simulink model "Mahendra_ev"  (R2024a)
settings: Solver=VariableStepAuto  StartTime=0.0  StopTime=100  RelTol=1e-3
undefined symbols (not defined in the file): magnitude
libraries: simulink_extras x1
settings Model: Creator=appu  LastModifiedBy=appu

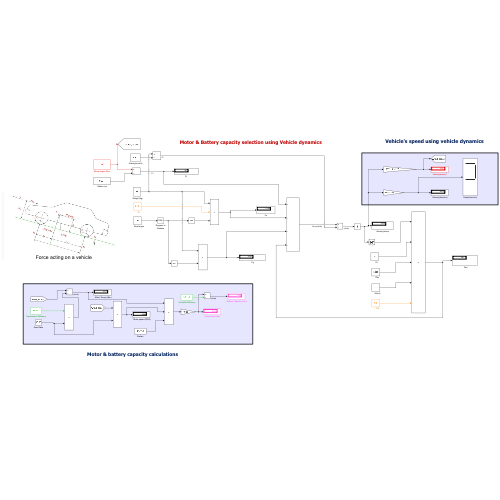
[thumbnail: Simulink's stored preview of the top-level diagram]
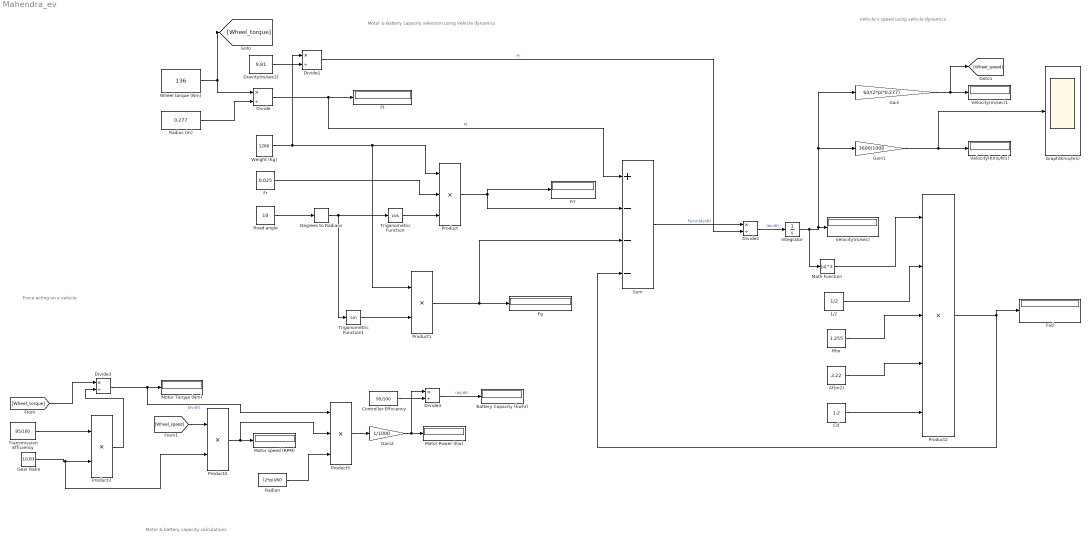
== system Mahendra_ev ==
  note: Force acting on a vehicle
  note: Vehicle's speed using vehicle dynamics
  note: Motor & battery capacity calculations
  note: Motor & Battery capacity selection using Vehicle dynamics
  "       Af(m2)" : Constant  Value=2.22
  "       Cd" : Constant  Value=1.2
  "      1/2" : Constant  Value=1/2
  "      Rho" : Constant  Value=1.255
  "      Road angle" : Constant  Value=10
  "     Fr" : Constant  Value=0.025
  "   Battery Capacity (kwhr)" : Display
  "   Fad" : Display
  "   Motor Torque (Nm)" : Display
  "   Motor speed (RPM)" : Display
  "   Weight (Kg)" : Constant  Value=1260
  "  Fg" : Display
  "  Motor Power (Kw)" : Display
  " Controller Efficiency" : Constant  Value=95/100
  " Frr" : Display
  " Gravity(m/sec2)" : Constant  Value=9.81
  " Radius (m)" : Constant  Value=0.277
  " Velocity(Kms/hrs)" : Display
  " Velocity(m/sec)" : Display
  " Velocity(m/sec)1" : Display
  Degrees to Radians : simulink_extras/Transformations/Degrees to Radians
  Divide{,1..4} (5 alike) : Product  Inputs=*/
  Ft : Display
  Gain : Gain  Gain=60/(2*pi*0.277)
  Gain1 : Gain  Gain=3600/1000
  Gain2 : Gain  Gain=1/1000
  Gear Ratio : Constant  Value=10.83
  Graph(Kms/hrs) : Scope
  Integrator : Integrator
  Math Function : Math  Operator=magnitude^2
  Product : Product  Inputs=3
  Product1 : Product
  Product2 : Product  Inputs=5
  Product3 : Product
  Product4 : Product
  Product5 : Product  Inputs=3
  Radian : Constant  Value=(2*pi)/60
  Sum : Sum  Inputs=+---
  Transmission Efficiency : Constant  Value=85/100
  Trigonometric Function : Trigonometry  Operator=cos
  Trigonometric Function1 : Trigonometry
  Wheel torque (Nm) : Constant  Value=136
  wires:
  Wheel torque (Nm)/1 -> [Wheel_torque], Divide/1
  " Radius (m)"/1 -> Divide/2
  "      Road angle"/1 -> Degrees to Radians/1
  Degrees to Radians/1 -> Trigonometric Function1/1, Trigonometric Function/1
  Trigonometric Function/1 -> Product/3
  "     Fr"/1 -> Product/2
  "   Weight (Kg)"/1 -> Product1/1, Product/1, Divide1/1
  Divide/1 -> Sum/1, Ft/1  "Ft"
  Product/1 -> Sum/2, " Frr"/1
  " Gravity(m/sec2)"/1 -> Divide1/2
  Sum/1 -> Divide2/1  "Fa=m(dv/dt)"
  Divide1/1 -> Divide2/2  "Ft"
  Divide2/1 -> Integrator/1  "(dv/dt)"
  Integrator/1 -> Math Function/1, Gain1/1, Gain/1, " Velocity(m/sec)"/1
  Math Function/1 -> Product2/1
  "      1/2"/1 -> Product2/2
  "      Rho"/1 -> Product2/3
  "       Af(m2)"/1 -> Product2/4
  "       Cd"/1 -> Product2/5
  Gain/1 -> [Wheel_speed], " Velocity(m/sec)1"/1
  Gain1/1 -> Graph(Kms/hrs)/1, " Velocity(Kms/hrs)"/1
  Product2/1 -> Sum/4, "   Fad"/1
  Transmission Efficiency/1 -> Product3/1
  Gear Ratio/1 -> Product4/2, Product3/2
  [Wheel_torque] -> Divide3/1
  Product3/1 -> Divide3/2
  [Wheel_speed] -> Product4/1
  Divide3/1 -> Product5/1, "   Motor Torque (Nm)"/1  "(dv/dt)"
  Product4/1 -> Product5/2, "   Motor speed (RPM)"/1
  Radian/1 -> Product5/3
  Product5/1 -> Gain2/1
  Gain2/1 -> Divide4/1, "  Motor Power (Kw)"/1
  " Controller Efficiency"/1 -> Divide4/2
  Divide4/1 -> "   Battery Capacity (kwhr)"/1  "(dv/dt)"
  Trigonometric Function1/1 -> Product1/2
  Product1/1 -> Sum/3, "  Fg"/1
